simulink model "SAR_Simulation"  (R2019a)
settings: Solver=VariableStepAuto  StartTime=0.0  StopTime=10.0  RelTol=1e-3
libraries: dspsigops x4, simulink x1
settings Model: Creator=CSP  LastModifiedBy=CSP

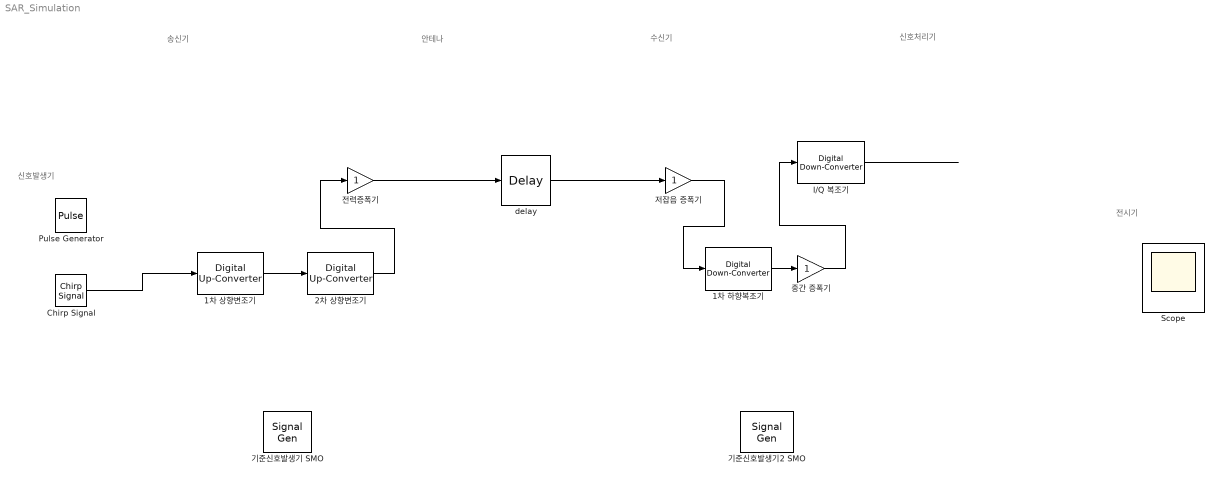
== system SAR_Simulation ==
  note: 안테나
  note: 신호처리기
  note: 수신기
  note: 송신기
  note: 전시기
  note: 신호발생기
  1차 상향변조기 : dspsigops/Digital Up-Converter  InterpolationFactor=100  MinimumOrderDesign=on  FirstFilterOrder=10  SecondFilterOrder=12  NumCICSections=3  Bandwidth=200000  StopbandFrequencySource=Auto  StopbandFrequency=150000  PassbandRipple=0.1  StopbandAttenuation=60  Oscillator=Sine wave  CenterFrequency=14e6  NumAccumulatorBits=16  NumQuantizedAccumulatorBits=12  Dither=on  NumDitherBits=4  InheritSampleRate=off  SampleRate=300000  SimulateUsing=Code generation  outputMin=[]  outputMax=[]
      settings: SourceProductName=DSP System Toolbox  SourceProductBaseCode=DS
  1차 하향복조기 : dspsigops/Digital Down-Converter  DecimationFactor=100  MinimumOrderDesign=on  NumCICSections=3  SecondFilterOrder=12  ThirdFilterOrder=10  Bandwidth=200000  StopbandFrequencySource=Auto  StopbandFrequency=150000  PassbandRipple=0.1  StopbandAttenuation=60  Oscillator=Sine wave  CenterFrequency=14e6  NumAccumulatorBits=16  NumQuantizedAccumulatorBits=12  Dither=on  NumDitherBits=4  InheritSampleRate=off  SampleRate=30000000  SimulateUsing=Code generation  outputMin=[]  outputMax=[]
      settings: SourceProductName=DSP System Toolbox  SourceProductBaseCode=DS
  2차 상향변조기 : dspsigops/Digital Up-Converter  InterpolationFactor=100  MinimumOrderDesign=on  FirstFilterOrder=10  SecondFilterOrder=12  NumCICSections=3  Bandwidth=200000  StopbandFrequencySource=Auto  StopbandFrequency=150000  PassbandRipple=0.1  StopbandAttenuation=60  Oscillator=Sine wave  CenterFrequency=14e6  NumAccumulatorBits=16  NumQuantizedAccumulatorBits=12  Dither=on  NumDitherBits=4  InheritSampleRate=off  SampleRate=300000  SimulateUsing=Code generation  outputMin=[]  outputMax=[]
      settings: SourceProductName=DSP System Toolbox  SourceProductBaseCode=DS
  "Chirp Signal " : simulink/Sources/Chirp Signal  f1=0.1  T=100  f2=1
  I/Q 복조기 : dspsigops/Digital Down-Converter  DecimationFactor=100  MinimumOrderDesign=on  NumCICSections=3  SecondFilterOrder=12  ThirdFilterOrder=10  Bandwidth=200000  StopbandFrequencySource=Auto  StopbandFrequency=150000  PassbandRipple=0.1  StopbandAttenuation=60  Oscillator=Sine wave  CenterFrequency=14e6  NumAccumulatorBits=16  NumQuantizedAccumulatorBits=12  Dither=on  NumDitherBits=4  InheritSampleRate=off  SampleRate=30000000  SimulateUsing=Code generation  outputMin=[]  outputMax=[]
      settings: SourceProductName=DSP System Toolbox  SourceProductBaseCode=DS
  "Pulse Generator " : DiscretePulseGenerator  PulseType=Time based  Period=10  PulseWidth=5
  "Scope " : Scope  NumInputPorts=2
  delay : TransportDelay
  기준신호발생기 SMO : SignalGenerator  Units=rad/sec
  기준신호발생기2 SMO : SignalGenerator  Units=rad/sec
  저잡음 증폭기 : Gain
  전력증폭기 : Gain
  중간 증폭기 : Gain
  wires:
  1차 상향변조기/1 -> 2차 상향변조기/1
  2차 상향변조기/1 -> 전력증폭기/1
  1차 하향복조기/1 -> 중간 증폭기/1
  저잡음 증폭기/1 -> 1차 하향복조기/1
  중간 증폭기/1 -> I/Q 복조기/1
  "Chirp Signal "/1 -> 1차 상향변조기/1
  전력증폭기/1 -> delay/1
  delay/1 -> 저잡음 증폭기/1
  I/Q 복조기/1 -> ?
